simulink model "generic"  (Simulink 10.2)
settings: Solver=ode45  StartTime=0.0  StopTime=inf  RelTol=1e-3  EnableMultiTasking=on
values from neighbouring files (symbols this model uses):
  I = 5000    [run_simulation.m]
  kappa_ref = 0.1    [run_simulation.m]
  N = 5    [kmpc_yalmip.m]    (also in kmpc_yalmip_adaptive.m; run_simulation.m = 4)
  P = 2500    [run_simulation.m]
  R = 0.318    [run_simulation.m]
  Tmax = 250    [run_simulation.m]
  Ts = 2e-3    (= 0.002)    [kmpc_yalmip.m]    (also in kmpc_yalmip_adaptive.m; run_simulation.m)
  w0 = 4.5    [run_simulation.m]
undefined symbols (not defined in the file or in its folder): DiscIntNeverNeededParam
libraries: CarMaker4SL x18, simulink x8, pid_lib x2
(part 3 of 3)

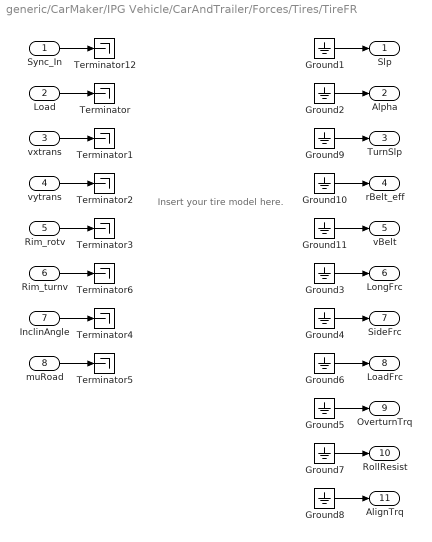
== system generic/CarMaker/IPG Vehicle/CarAndTrailer/Forces/Tires/TireFR ==
  note: Insert your tire model here.
  Sync_In : Inport
  Load : Inport  Port=2
  vxtrans : Inport  Port=3
  vytrans : Inport  Port=4
  Rim_rotv : Inport  Port=5
  Rim_turnv : Inport  Port=6
  InclinAngle : Inport  Port=7
  muRoad : Inport  Port=8
  Ground{1..11} (11 alike) : Ground
  Terminator{,1..6,12} (8 alike) : Terminator
  Slp : Outport  VectorParamsAs1DForOutWhenUnconnected=off
  Alpha : Outport  Port=2  VectorParamsAs1DForOutWhenUnconnected=off
  TurnSlp : Outport  Port=3  VectorParamsAs1DForOutWhenUnconnected=off
  rBelt_eff : Outport  Port=4  VectorParamsAs1DForOutWhenUnconnected=off
  vBelt : Outport  Port=5  VectorParamsAs1DForOutWhenUnconnected=off
  LongFrc : Outport  Port=6  VectorParamsAs1DForOutWhenUnconnected=off
  SideFrc : Outport  Port=7  VectorParamsAs1DForOutWhenUnconnected=off
  LoadFrc : Outport  Port=8  VectorParamsAs1DForOutWhenUnconnected=off
  OverturnTrq : Outport  Port=9  VectorParamsAs1DForOutWhenUnconnected=off
  RollResist : Outport  Port=10  VectorParamsAs1DForOutWhenUnconnected=off
  AlignTrq : Outport  Port=11  VectorParamsAs1DForOutWhenUnconnected=off
  wires:
  Ground11/1 -> vBelt/1
  Ground10/1 -> rBelt_eff/1
  Ground9/1 -> TurnSlp/1
  Rim_turnv/1 -> Terminator6/1
  Sync_In/1 -> Terminator12/1
  Ground2/1 -> Alpha/1
  Ground3/1 -> LongFrc/1
  Ground4/1 -> SideFrc/1
  Ground5/1 -> OverturnTrq/1
  vxtrans/1 -> Terminator1/1
  vytrans/1 -> Terminator2/1
  Rim_rotv/1 -> Terminator3/1
  InclinAngle/1 -> Terminator4/1
  muRoad/1 -> Terminator5/1
  Load/1 -> Terminator/1
  Ground1/1 -> Slp/1
  Ground6/1 -> LoadFrc/1
  Ground7/1 -> RollResist/1
  Ground8/1 -> AlignTrq/1

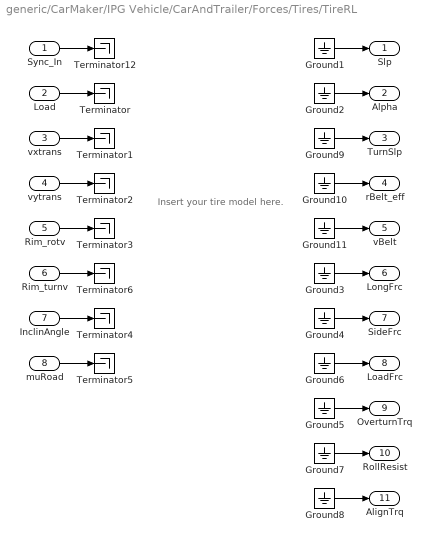
== system generic/CarMaker/IPG Vehicle/CarAndTrailer/Forces/Tires/TireRL ==
  note: Insert your tire model here.
  Sync_In : Inport
  Load : Inport  Port=2
  vxtrans : Inport  Port=3
  vytrans : Inport  Port=4
  Rim_rotv : Inport  Port=5
  Rim_turnv : Inport  Port=6
  InclinAngle : Inport  Port=7
  muRoad : Inport  Port=8
  Ground{1..11} (11 alike) : Ground
  Terminator{,1..6,12} (8 alike) : Terminator
  Slp : Outport  VectorParamsAs1DForOutWhenUnconnected=off
  Alpha : Outport  Port=2  VectorParamsAs1DForOutWhenUnconnected=off
  TurnSlp : Outport  Port=3  VectorParamsAs1DForOutWhenUnconnected=off
  rBelt_eff : Outport  Port=4  VectorParamsAs1DForOutWhenUnconnected=off
  vBelt : Outport  Port=5  VectorParamsAs1DForOutWhenUnconnected=off
  LongFrc : Outport  Port=6  VectorParamsAs1DForOutWhenUnconnected=off
  SideFrc : Outport  Port=7  VectorParamsAs1DForOutWhenUnconnected=off
  LoadFrc : Outport  Port=8  VectorParamsAs1DForOutWhenUnconnected=off
  OverturnTrq : Outport  Port=9  VectorParamsAs1DForOutWhenUnconnected=off
  RollResist : Outport  Port=10  VectorParamsAs1DForOutWhenUnconnected=off
  AlignTrq : Outport  Port=11  VectorParamsAs1DForOutWhenUnconnected=off
  wires:
  Ground11/1 -> vBelt/1
  Ground10/1 -> rBelt_eff/1
  Ground9/1 -> TurnSlp/1
  Rim_turnv/1 -> Terminator6/1
  Sync_In/1 -> Terminator12/1
  Ground2/1 -> Alpha/1
  Ground3/1 -> LongFrc/1
  Ground4/1 -> SideFrc/1
  Ground5/1 -> OverturnTrq/1
  vxtrans/1 -> Terminator1/1
  vytrans/1 -> Terminator2/1
  Rim_rotv/1 -> Terminator3/1
  InclinAngle/1 -> Terminator4/1
  muRoad/1 -> Terminator5/1
  Load/1 -> Terminator/1
  Ground1/1 -> Slp/1
  Ground6/1 -> LoadFrc/1
  Ground7/1 -> RollResist/1
  Ground8/1 -> AlignTrq/1

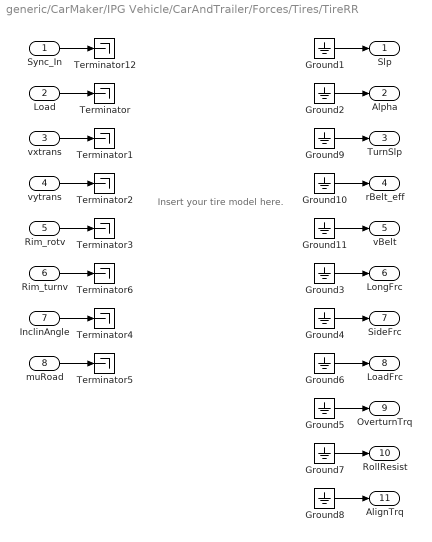
== system generic/CarMaker/IPG Vehicle/CarAndTrailer/Forces/Tires/TireRR ==
  note: Insert your tire model here.
  Sync_In : Inport
  Load : Inport  Port=2
  vxtrans : Inport  Port=3
  vytrans : Inport  Port=4
  Rim_rotv : Inport  Port=5
  Rim_turnv : Inport  Port=6
  InclinAngle : Inport  Port=7
  muRoad : Inport  Port=8
  Ground{1..11} (11 alike) : Ground
  Terminator{,1..6,12} (8 alike) : Terminator
  Slp : Outport  VectorParamsAs1DForOutWhenUnconnected=off
  Alpha : Outport  Port=2  VectorParamsAs1DForOutWhenUnconnected=off
  TurnSlp : Outport  Port=3  VectorParamsAs1DForOutWhenUnconnected=off
  rBelt_eff : Outport  Port=4  VectorParamsAs1DForOutWhenUnconnected=off
  vBelt : Outport  Port=5  VectorParamsAs1DForOutWhenUnconnected=off
  LongFrc : Outport  Port=6  VectorParamsAs1DForOutWhenUnconnected=off
  SideFrc : Outport  Port=7  VectorParamsAs1DForOutWhenUnconnected=off
  LoadFrc : Outport  Port=8  VectorParamsAs1DForOutWhenUnconnected=off
  OverturnTrq : Outport  Port=9  VectorParamsAs1DForOutWhenUnconnected=off
  RollResist : Outport  Port=10  VectorParamsAs1DForOutWhenUnconnected=off
  AlignTrq : Outport  Port=11  VectorParamsAs1DForOutWhenUnconnected=off
  wires:
  Ground11/1 -> vBelt/1
  Ground10/1 -> rBelt_eff/1
  Ground9/1 -> TurnSlp/1
  Rim_turnv/1 -> Terminator6/1
  Sync_In/1 -> Terminator12/1
  Ground2/1 -> Alpha/1
  Ground3/1 -> LongFrc/1
  Ground4/1 -> SideFrc/1
  Ground5/1 -> OverturnTrq/1
  vxtrans/1 -> Terminator1/1
  vytrans/1 -> Terminator2/1
  Rim_rotv/1 -> Terminator3/1
  InclinAngle/1 -> Terminator4/1
  muRoad/1 -> Terminator5/1
  Load/1 -> Terminator/1
  Ground1/1 -> Slp/1
  Ground6/1 -> LoadFrc/1
  Ground7/1 -> RollResist/1
  Ground8/1 -> AlignTrq/1

== matlab function CarMaker/Traction control/ControllerFL/NMPC/MATLAB Function ==
  data: e_int input double; current_state input double; ocp_state output double; R parameter double
function ocp_state = create_ocp_state(e_int,current_state, R)
    v = current_state(1);
    w = current_state(2);
    ocp_state = [w*R-v; w; e_int];
end

== matlab function CarMaker/Traction control/MATLAB Function ==
  data: u input double; y output double
function y = scalar2array(u)
y = repelem(u,4,1);

== matlab function CarMaker/Traction control/ControllerFL/NMPC/MATLAB Function2 ==
  data: u input double; y output double; N parameter double
function y = repeat_elements(u, N)
    y = repmat(u,N,1);
end

== matlab function CarMaker/Traction control/ControllerFR/NMPC/MATLAB Function ==
  data: e_int input double; current_state input double; ocp_state output double; R parameter double
function ocp_state = create_ocp_state(e_int,current_state, R)
    v = current_state(1);
    w = current_state(2);
    ocp_state = [w*R-v; w; e_int];
end

== matlab function CarMaker/Traction control/ControllerFL/NMPC/MATLAB Function4 ==
  data: u input double; y output double; N parameter double
function y = repeat_elements(u, N)
    y = repmat(u,N,1);
end

== matlab function CarMaker/Traction control/ControllerFL/NMPC/e_int_dot ==
  data: current_state input double; e_int_dot output double; kappa_ref parameter double; R parameter double
function e_int_dot = fcn(current_state,kappa_ref,R)
e_int_dot = kappa_ref - current_state(3);
% v = current_state(1);
% w = current_state(2);
% s = w*R - v;
% epsilon = 0*1e-3;
% e_int_dot = kappa_ref - s/(w*R+epsilon);
end

== matlab function CarMaker/Traction control/ControllerFL/NMPC/MATLAB Function3 ==
  data: current_state input double; s_ref output double; s output double; kappa_ref parameter double; R parameter double
function [s_ref,s] = fcn(current_state,kappa_ref, R)
    v = current_state(1);
    w = current_state(2);
    s = w*R - v;
    s_ref = kappa_ref*w*R;
end

== matlab function CarMaker/Traction control/ControllerFR/NMPC/MATLAB Function2 ==
  data: u input double; y output double; N parameter double
function y = repeat_elements(u, N)
    y = repmat(u,N,1);
end

== matlab function CarMaker/Traction control/ControllerFR/NMPC/MATLAB Function4 ==
  data: u input double; y output double; N parameter double
function y = repeat_elements(u, N)
    y = repmat(u,N,1);
end

== matlab function CarMaker/Traction control/ControllerFL/NMPC/MATLAB Function1 ==
  data: hu input double; alles_gut output double; hl input double; x0 input double; xinit input double; p input double; N parameter double; exitflag input double; zopt input double; t input double
function alles_gut = check_solver_output(hu,hl,x0,xinit,p,N,exitflag,zopt,t)
if exitflag ~= 1
    disp(['problem at t=',sprintf('%.3f',t),': exitflag = ',sprintf('%.0f',exitflag)])
    zopt;
end
% https://forces.embotech.com/Documentation/faq/index.html#issues-when-running-a-generated-solver
coder.extrinsic('nmpc_dynamics','nmpc_inequalities','nmpc_objective')
alles_gut = 0; hu; hl; xinit;
jj = 1;
nvar = 4;
c = nan(3,1);
jacc = nan(3,4);
ineq = nan;
jacineq = nan(1,4);
obj = nan;
gradobj = nan(4,1);
for stage = 1:N-1
    z = x0(jj:(jj+nvar-1));
    [c, jacc] = nmpc_dynamics(z, p, stage);
    [ineq, jacineq] = nmpc_inequalities(z, p, stage);
    [obj, gradobj] = nmpc_objective(z, p, stage);
    assert(~any(isnan(c) | isinf(c), 'all'), 'Encountered NaNs or Infs in c at stage %d', stage);
    assert(~any(isnan(jacc) | isinf(jacc), 'all'), 'Encountered NaNs or Infs in jacc at stage %d', stage);
    assert(~any(isnan(ineq) | isinf(ineq), 'all'), 'Encountered NaNs or Infs in ineq at stage %d', stage);
    assert(~any(isnan(jacineq) | isinf(jacineq), 'all'), 'Encountered NaNs or Infs in jacineq at stage %d', stage);
    assert(~any(isnan(obj) | isinf(obj), 'all'), 'Encountered NaNs or Infs in obj at stage %d', stage);
    assert(~any(isnan(gradobj) | isinf(gradobj), 'all'), 'Encountered NaNs or Infs in gradobj at stage %d', stage);
    jj = jj + nvar;
end
alles_gut = 1;
end

== matlab function CarMaker/Traction control/ControllerFR/NMPC/e_int_dot ==
  data: current_state input double; e_int_dot output double; kappa_ref parameter double; R parameter double
function e_int_dot = fcn(current_state,kappa_ref,R)
e_int_dot = kappa_ref - current_state(3);
% v = current_state(1);
% w = current_state(2);
% s = w*R - v;
% epsilon = 0*1e-3;
% e_int_dot = kappa_ref - s/(w*R+epsilon);
end
